simulink model "Planta_controlada"  (R2024a)
settings: Solver=VariableStepAuto  StartTime=0.0  StopTime=8  RelTol=1e-3
undefined symbols (not defined in the file): DenZ, NumZ, Ts
libraries: slpidlib x1
settings Model: Creator=cesar  LastModifiedBy=cesar
settings DataIOCC: SaveFormat=StructureWithTime  SaveOutput=off  TimeSaveName=time  OutputSaveName=signals.values

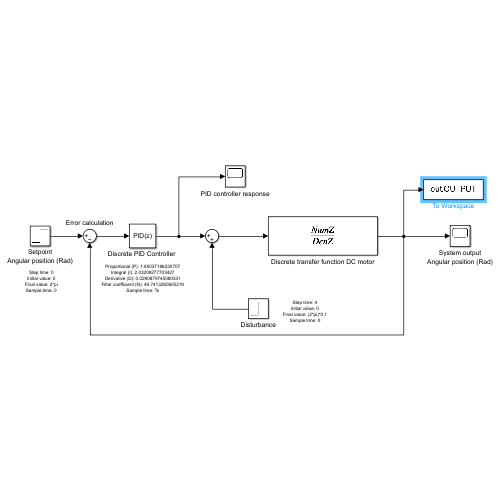
[thumbnail: Simulink's stored preview of the top-level diagram]
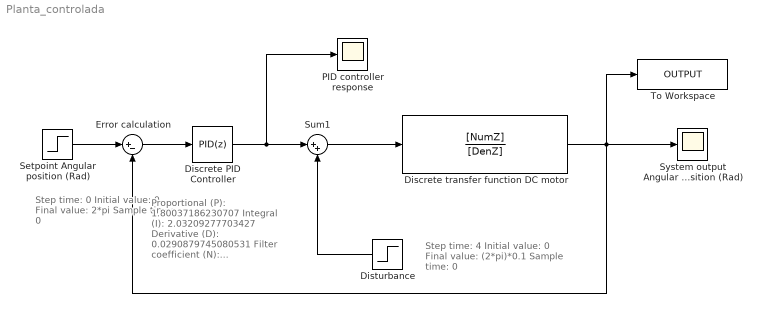
== system Planta_controlada ==
  note: Step time: 0
      | Initial value: 0
      | Final value: 2*pi
      | Sample time: 0
  note: Proportional (P): 1.80037186230707
      | Integral (I): 2.03209277703427
      | Derivative (D): 0.0290879745080531
      | Filter coefficient (N): 49.7413280605219
      | Sample time: Ts
  note: Step time: 4
      | Initial value: 0
      | Final value: (2*pi)*0.1
      | Sample time: 0
  "Discrete PID Controller " : slpidlib/PID Controller  Controller=PID  Form=Parallel  TimeDomain=Discrete-time  UseExternalTs=off  SampleTime=Ts  IntegratorMethod=Forward Euler  FilterMethod=Forward Euler  ControllerParametersSource=internal  P=1.80037186230707  I=2.03209277703427  UseKiTs=off  D=0.0290879745080531  UseExternalDerivativeSource=off  N=49.7413280605219  UseFilter=on  TunerSelectOption=Transfer Function Based (PID Tuner App)  InitialConditionSource=internal  InitialConditionForIntegrator=0  InitialConditionForFilter=0  DifferentiatorICPrevScaledInput=0  ExternalReset=none  TrackingMode=off  Kt=1  LimitOutput=off  SatLimitsSource=internal  UpperSaturationLimit=inf  LowerSaturationLimit=-inf  LinearizeAsGain=on  AntiWindupMode=none  Kb=1  LimitIntegrator=off  UpperIntegratorSaturationLimit=inf  LowerIntegratorSaturationLimit=-inf  POutMin=[]  POutMax=[]  IOutMin=[]  IOutMax=[]  DOutMin=[]  DOutMax=[]  NOutMin=[]  NOutMax=[]  SumOutMin=[]  SumOutMax=[]  SaturationOutMin=[]  SaturationOutMax=[]  PParamMin=[]  PParamMax=[]  IParamMin=[]  IParamMax=[]  DParamMin=[]  DParamMax=[]  NParamMin=[]  NParamMax=[]  KbParamMin=[]  KbParamMax=[]  KtParamMin=[]  KtParamMax=[]  KbOutMin=[]  KbOutMax=[]  KtOutMin=[]  KtOutMax=[]  IntegratorOutMin=[]  IntegratorOutMax=[]  FilterOutMin=[]  FilterOutMax=[]  SumI1OutMin=[]  SumI1OutMax=[]  SumI2OutMin=[]  SumI2OutMax=[]  SumI3OutMin=[]  SumI3OutMax=[]  SumI4OutMin=[]  SumI4OutMax=[]  SumDOutMin=[]  SumDOutMax=[]  DifferentiatorOutMin=[]  DifferentiatorOutMax=[]  FilterDiffOutCoefMin=[]  FilterDiffOutCoefMax=[]  ReciprocalOutMin=[]  ReciprocalOutMax=[]  SumDenOutMin=[]  SumDenOutMax=[]  SumNumOutMin=[]  SumNumOutMax=[]  DivideOutMin=[]  DivideOutMax=[]  UdiffTsProdOutMin=[]  UdiffTsProdOutMax=[]  NTsProdOutMin=[]  NTsProdOutMax=[]  UintegralTsProdOutMin=[]  UintegralTsProdOutMax=[]  UngainTsProdOutMin=[]  UngainTsProdOutMax=[]  ClampingZeroOutDataTypeStr=Inherit: Inherit via back propagation  ClampingZeroOutMin=[]  ClampingZeroOutMax=[]  FilterDenConstantOutDataTypeStr=Inherit: Inherit via back propagation  FilterDenConstantOutMin=[]  FilterDenConstantOutMax=[]  PCopyOutDataTypeStr=Inherit: Inherit via back propagation  PCopyOutMin=[]  PCopyOutMax=[]  NCopyOutDataTypeStr=Inherit: Inherit via back propagation  NCopyOutMin=[]  NCopyOutMax=[]  IntegratorContinuousStateAttributes=''  IntegratorStateMustResolveToSignalObject=off  IntegratorRTWStateStorageClass=Auto  FilterContinuousStateAttributes=''  FilterStateMustResolveToSignalObject=off  FilterRTWStateStorageClass=Auto  ParallelPVariant=InternalParameters  IdealPVariant=Disabled  IVariant=InternalParameters  DVariant=InternalParameters  IntegratorVariant=Discrete  SatVariant=Disabled  AWVariant=Passthrough  PCopyVariant=Disabled  TRVariant=Disabled  FdbkBlocksVariant=Forward  IdealPFdbkVariant=Disabled  SatFdbkVariant=Disabled  DerivativeFilterVariant=ForwardEulerFilter  NVariant=InternalParameters  NCopyVariant=Disabled  FilterICVariant=InternalICsFilter  IntegratorICVariant=InternalICs  ExternalResetVariant=Disabled  TRSumVariant=Passthrough  SumFdbkVariant=Disabled  SumVariant=Sum_PID  TsampFilterVariant=InternalTs  TsampNgainVariant=Passthrough  TsampIntegralVariant=Disabled_SignalSpec  ExternalSaturationOutDataTypeStr=Inherit: Same as second input  DerivativeSourceVariant=ErrorSignal
  Discrete transfer function DC motor : DiscreteTransferFcn  Numerator=[NumZ]  Denominator=[DenZ]  SampleTime=0.01
  Disturbance : Step  Time=4  After=(2*pi)*0.1  SampleTime=0
  Error calculation : Sum  Inputs=|+-
  PID controller response : Scope
  "Setpoint Angular position (Rad) " : Step  Time=0  After=2*pi  SampleTime=0
  Sum1 : Sum  Inputs=|++
  "System output Angular position (Rad) " : Scope
  To Workspace : ToWorkspace  VariableName=OUTPUT  SaveFormat=Structure With Time  SampleTime=-1
  wires:
  "Setpoint Angular position (Rad) "/1 -> Error calculation/1
  Discrete transfer function DC motor/1 -> To Workspace/1, "System output Angular position (Rad) "/1, Error calculation/2
  Error calculation/1 -> "Discrete PID Controller "/1
  "Discrete PID Controller "/1 -> PID controller response/1, Sum1/1
  Sum1/1 -> Discrete transfer function DC motor/1
  Disturbance/1 -> Sum1/2
